simulink model "SE17"  (R2021a)
settings: Solver=FixedStepAuto  StartTime=0.0  StopTime=20  FixedStep=.01  RelTol=1e-3
undefined symbols (not defined in the file or in its folder): Ion, Li, r_c, r_D, u_ce0, u_D0
libraries: Lib_EMTAT x26, pid_lib x5
(part 2 of 2)

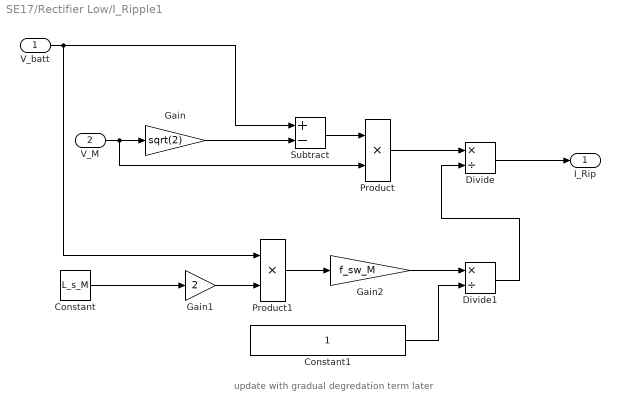
== system SE17/Rectifier Low/I_Ripple1 ==
  note: update with gradual degredation term later
  V_batt : Inport
  "V_M " : Inport  Port=2
  Constant : Constant  Value=L_s_M
  Constant1 : Constant
  Divide : Product  Inputs=*/
  Divide1 : Product  Inputs=*/
  Gain : Gain  Gain=sqrt(2)
  Gain1 : Gain  Gain=2
  Gain2 : Gain  Gain=f_sw_M
  Product : Product
  Product1 : Product
  Subtract : Sum  Inputs=+-
  I_Rip : Outport  VectorParamsAs1DForOutWhenUnconnected=off
  wires:
  Divide1/1 -> Divide/2
  Constant1/1 -> Divide1/2
  Gain2/1 -> Divide1/1
  "V_M "/1 -> Product/2, Gain/1
  Gain/1 -> Subtract/2
  V_batt/1 -> Subtract/1, Product1/1
  Subtract/1 -> Product/1
  Product/1 -> Divide/1
  Constant/1 -> Gain1/1
  Gain1/1 -> Product1/2
  Product1/1 -> Gain2/1
  Divide/1 -> I_Rip/1

== system SE17/Rectifier Low/P_out_gen ==
  I (RMS) : Inport
  V_s (RMS) : Inport  Port=2
  PF : Inport  Port=3
  Gain : Gain  Gain=sqrt(3)
  Product : Product  Inputs=3
  P_out_gen : Outport  VectorParamsAs1DForOutWhenUnconnected=off
  wires:
  I (RMS)/1 -> Product/2
  PF/1 -> Product/3
  V_s (RMS)/1 -> Product/1
  Gain/1 -> P_out_gen/1
  Product/1 -> Gain/1

== system SE17/Rectifier Low/mVal ==
  V_s : Inport
  V_batt : Inport  Port=2
  Divide : Product  Inputs=*/
  Gain : Gain  Gain=sqrt(2)
  m : Outport  VectorParamsAs1DForOutWhenUnconnected=off
  wires:
  Divide/1 -> m/1
  V_s/1 -> Gain/1
  Gain/1 -> Divide/1
  V_batt/1 -> Divide/2
